simulink model "EST_Modified_Copy"  (R2023a)
settings: Solver=FixedStepAuto  StartTime=0.0  StopTime=stopt  FixedStep=deltat  MaxStep=0.05  RelTol=1e-3
InitFcn:
  | clear all;
  | close all;
  | clc;
  | 
  | % add the data and script directories
  | addpath('data','scripts');
  | 
  | % load the constants (units)
  | constants;
  | 
  | % load the simulation parameters
  | preprocessing;
StopFcn:
  | postprocessing;
values from neighbouring files (symbols this model uses):
  aDemandTransport = 0.03    [preprocessing.m]
  aExtraction = 0.80    (= 0.8)    [preprocessing.m]
  aHeatCompressor = 0.07    [preprocessing.m]
  aHeatGenerator = 0.1    [preprocessing.m]
  aInjection = 0.15    [preprocessing.m]
  aSupplyTransport = 0.03    [preprocessing.m]
  bHeatExchanger = 0.001    [preprocessing.m]
  bStorage = 0.000/unit("s")    [preprocessing.m]
  EStorageInitial = 0.000*unit("kWh")    [preprocessing.m]
  EStorageMax = (25/3)*unit("kWh")    [preprocessing.m]
  EStorageMin = 0.000*unit("kWh")    [preprocessing.m]
  HeatExchangerInitial = 0    [preprocessing.m]
settings Model: Creator=joche  LastModifiedBy=20221247
settings DataIOCC: SaveFormat=Array  SaveOutput=off  ReturnWorkspaceOutputs=off
settings OptimizationCC: ReuseModelBlockBuffer=off
settings ModelReferenceCC: EnableRefExpFcnMdlSchedulingChecks=on

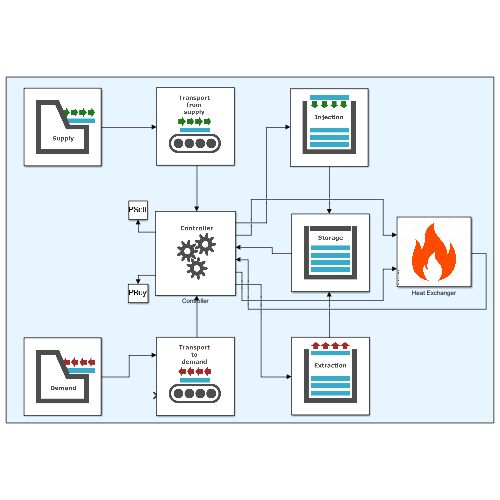
[thumbnail: Simulink's stored preview of the top-level diagram]
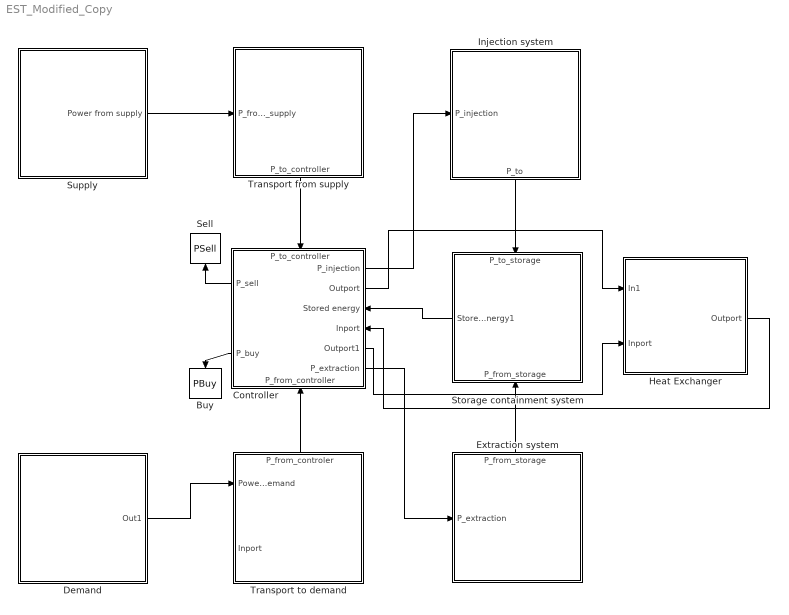
== system EST_Modified_Copy ==
  Buy : ToWorkspace  VariableName=PBuy  SampleTime=-1
  Controller : Subsystem
      settings: PortSchema="{\"entries\":[{\"content\":{\"sides\":[{\"content\":{\"connectorIds\":[\"Out5\",\"Out6\"]},\"type\":\"ConnectorPlacement.EquallySpacedRectSide\",\"uuid\":\"4daf33ce-c96a-4783-b5c4-228eed953e01\"},{\"content\":{\"connectorIds\":[\"Out1\",\"Out2\",\"In3\",\"In4\",\"Out3\",\"Out4\"],\"side\":\"RIGHT\"},\"type\":\"ConnectorPlacement.EquallySpacedRectSide\",\"uuid\":\"e9942e50-8467-4af8-b79b-80636cbc76e5\"},{\"content\":{\"connectorIds\":[\"In1\"],\"side\":\"TOP\"},\"type\":\"ConnectorPlacement.EquallySpacedRectSide\",\"uuid\":\"f315e931-d69b-4751-b712-f89c6c81baeb\"},{\"content\":{\"connectorIds\":[\"In2\"],\"side\":\"BOTTOM\"},\"type\":\"ConnectorPlacement.EquallySpacedRectSide\",\"uuid\":\"44715ee6-5cd5-4669-bcb9-5ed7c869bdb3\"}]},\"type\":\"ConnectorPlacement.EquallySpacedConnector\",\"uuid\":\"fff48899-944b-4064-b7d7-ecc12144fb48\"}],\"packageUris\":[\"http://schema.mathworks.com/mf0/Connector/R2020b\"],\"version\":\"1.0\"}"
      mask Display: image('$imagefile'); % Use "Edit Image" on toolstrip to change.
  Demand : Subsystem
      mask Display: image('$imagefile'); % Use "Edit Image" on toolstrip to change.
  Extraction system : Subsystem
      settings: PortSchema="{\"entries\":[{\"content\":{\"sides\":[{\"content\":{},\"type\":\"ConnectorPlacement.EquallySpacedRectSide\",\"uuid\":\"05c5933d-55fc-4e06-853f-fc26d42905f9\"},{\"content\":{\"connectorIds\":[\"In1\"],\"side\":\"RIGHT\"},\"type\":\"ConnectorPlacement.EquallySpacedRectSide\",\"uuid\":\"327426c5-31d5-498b-a2bd-83e49353408c\"},{\"content\":{\"side\":\"TOP\"},\"type\":\"ConnectorPlacement.EquallySpacedRectSide\",\"uuid\":\"55306cf3-a3de-4385-a5ae-b8600ecdd5a2\"},{\"content\":{\"connectorIds\":[\"Out1\"],\"side\":\"BOTTOM\"},\"type\":\"ConnectorPlacement.EquallySpacedRectSide\",\"uuid\":\"08fcc9c3-40d3-4ac6-b914-dfeef6039ffb\"}]},\"type\":\"ConnectorPlacement.EquallySpacedConnector\",\"uuid\":\"cb35d5ba-e8c6-462c-b7b2-fe8356d4b0a1\"}],\"packageUris\":[\"http://schema.mathworks.com/mf0/Connector/R2020b\"],\"version\":\"1.0\"}"
      mask Display: image('$imagefile'); % Use "Edit Image" on toolstrip to change.
  Heat Exchanger : Subsystem
      mask Display: image('Heat Exchanger Icon.jpg'); % Use "Edit Image" on toolstrip to change.
  Injection system : Subsystem
      settings: PortSchema="{\"entries\":[{\"content\":{\"sides\":[{\"content\":{},\"type\":\"ConnectorPlacement.EquallySpacedRectSide\",\"uuid\":\"05c5933d-55fc-4e06-853f-fc26d42905f9\"},{\"content\":{\"connectorIds\":[\"In1\"],\"side\":\"RIGHT\"},\"type\":\"ConnectorPlacement.EquallySpacedRectSide\",\"uuid\":\"327426c5-31d5-498b-a2bd-83e49353408c\"},{\"content\":{\"connectorIds\":[\"Out1\"],\"side\":\"TOP\"},\"type\":\"ConnectorPlacement.EquallySpacedRectSide\",\"uuid\":\"55306cf3-a3de-4385-a5ae-b8600ecdd5a2\"},{\"content\":{\"side\":\"BOTTOM\"},\"type\":\"ConnectorPlacement.EquallySpacedRectSide\",\"uuid\":\"08fcc9c3-40d3-4ac6-b914-dfeef6039ffb\"}]},\"type\":\"ConnectorPlacement.EquallySpacedConnector\",\"uuid\":\"cb35d5ba-e8c6-462c-b7b2-fe8356d4b0a1\"}],\"packageUris\":[\"http://schema.mathworks.com/mf0/Connector/R2020b\"],\"version\":\"1.0\"}"
      mask Display: image('$imagefile'); % Use "Edit Image" on toolstrip to change.
  Sell : ToWorkspace  VariableName=PSell  SampleTime=-1
  Storage containment system : Subsystem
      settings: PortSchema="{\"entries\":[{\"content\":{\"sides\":[{\"content\":{\"connectorIds\":[\"Out1\"]},\"type\":\"ConnectorPlacement.EquallySpacedRectSide\",\"uuid\":\"0ba48424-33b9-4934-970f-64fe5d8b070e\"},{\"content\":{\"connectorIds\":[],\"side\":\"RIGHT\"},\"type\":\"ConnectorPlacement.EquallySpacedRectSide\",\"uuid\":\"9cde340f-8f39-4499-9a12-5e1623737660\"},{\"content\":{\"connectorIds\":[\"In1\"],\"side\":\"TOP\"},\"type\":\"ConnectorPlacement.EquallySpacedRectSide\",\"uuid\":\"2af8db04-7fd0-4902-8637-8dc00edb4598\"},{\"content\":{\"connectorIds\":[\"In2\"],\"side\":\"BOTTOM\"},\"type\":\"ConnectorPlacement.EquallySpacedRectSide\",\"uuid\":\"e21ea806-d777-41a3-a53f-556fae66854b\"}]},\"type\":\"ConnectorPlacement.EquallySpacedConnector\",\"uuid\":\"4e2ddb36-4db3-4ab4-858b-ebb8ccefeb1f\"}],\"packageUris\":[\"http://schema.mathworks.com/mf0/Connector/R2020b\"],\"version\":\"1.0\"}"
      mask Display: image('$imagefile'); % Use "Edit Image" on toolstrip to change.
  Supply : Subsystem
      mask Display: image('$imagefile'); % Use "Edit Image" on toolstrip to change.
  Transport from supply : Subsystem
      settings: PortSchema="{\"entries\":[{\"content\":{\"sides\":[{\"content\":{\"connectorIds\":[\"In1\"]},\"type\":\"ConnectorPlacement.EquallySpacedRectSide\",\"uuid\":\"31329006-3d36-4d93-9c44-7503a515d397\"},{\"content\":{\"connectorIds\":[],\"side\":\"RIGHT\"},\"type\":\"ConnectorPlacement.EquallySpacedRectSide\",\"uuid\":\"aba139c7-f9b6-4881-a56b-a4cbbedacd88\"},{\"content\":{\"connectorIds\":[],\"side\":\"TOP\"},\"type\":\"ConnectorPlacement.EquallySpacedRectSide\",\"uuid\":\"e683eb73-7a35-4160-9c39-da83856a6278\"},{\"content\":{\"connectorIds\":[\"Out1\"],\"side\":\"BOTTOM\"},\"type\":\"ConnectorPlacement.EquallySpacedRectSide\",\"uuid\":\"1170dd18-447c-437f-9043-6812c2877331\"}]},\"type\":\"ConnectorPlacement.EquallySpacedConnector\",\"uuid\":\"804af608-1d70-444f-af69-e05f19bf98f3\"}],\"packageUris\":[\"http://schema.mathworks.com/mf0/Connector/R2020b\"],\"version\":\"1.0\"}"
      mask Display: image('$imagefile'); % Use "Edit Image" on toolstrip to change.
  Transport to demand : Subsystem
      settings: PortSchema="{\"entries\":[{\"content\":{\"sides\":[{\"content\":{\"connectorIds\":[\"In1\",\"In2\"]},\"type\":\"ConnectorPlacement.EquallySpacedRectSide\",\"uuid\":\"31329006-3d36-4d93-9c44-7503a515d397\"},{\"content\":{\"side\":\"RIGHT\"},\"type\":\"ConnectorPlacement.EquallySpacedRectSide\",\"uuid\":\"aba139c7-f9b6-4881-a56b-a4cbbedacd88\"},{\"content\":{\"connectorIds\":[\"Out1\"],\"side\":\"TOP\"},\"type\":\"ConnectorPlacement.EquallySpacedRectSide\",\"uuid\":\"e683eb73-7a35-4160-9c39-da83856a6278\"},{\"content\":{\"side\":\"BOTTOM\"},\"type\":\"ConnectorPlacement.EquallySpacedRectSide\",\"uuid\":\"c378138f-7233-4483-870c-40a69b3495ee\"}]},\"type\":\"ConnectorPlacement.EquallySpacedConnector\",\"uuid\":\"804af608-1d70-444f-af69-e05f19bf98f3\"}],\"packageUris\":[\"http://schema.mathworks.com/mf0/Connector/R2020b\"],\"version\":\"1.0\"}"
      mask Display: image('$imagefile'); % Use "Edit Image" on toolstrip to change.
  wires:
  Supply/1(Power from supply) -> Transport from supply/1(P_from_supply)
  Transport from supply/1(P_to_controller) -> Controller/1(P_to_controller)
  Transport to demand/1(P_from_controler) -> Controller/2(P_from_controller)
  Demand/1(Out1) -> Transport to demand/1(Power to demand)
  Controller/5(P_sell) -> Sell/1
  Controller/4(P_extraction) -> Extraction system/1(P_extraction)
  Injection system/1(P_to) -> Storage containment system/1(P_to_storage)
  Extraction system/1(P_from_storage) -> Storage containment system/2(P_from_storage)
  Storage containment system/1(Stored energy1) -> Controller/3(Stored energy)
  Controller/1(P_injection) -> Injection system/1(P_injection)
  Controller/6(P_buy) -> Buy/1
  Controller/2(Outport) -> Heat Exchanger/1(In1)
  Controller/3(Outport1) -> Heat Exchanger/2(Inport)
  Heat Exchanger/1(Outport) -> Controller/4(Inport)

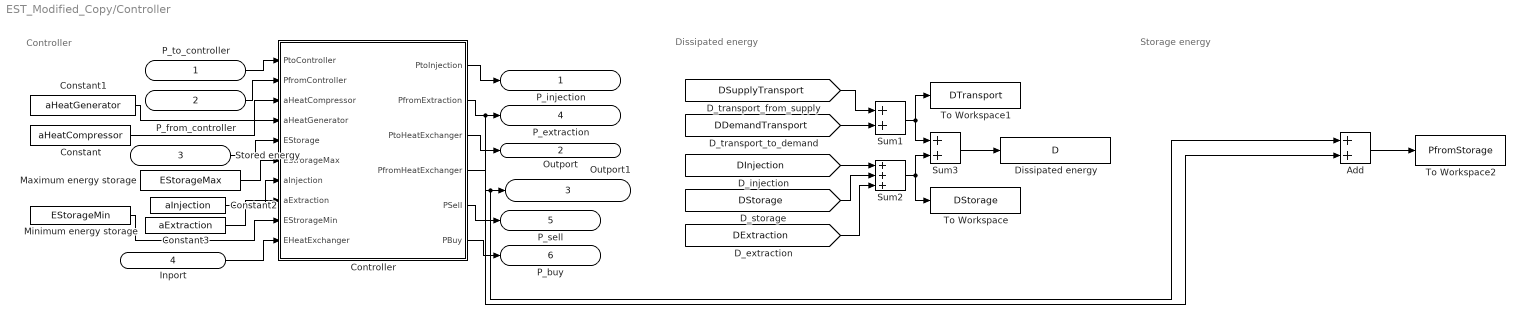
== system EST_Modified_Copy/Controller ==
  note: Dissipated energy
  note: Controller
  note: Storage energy
  P_to_controller : Inport
  P_from_controller : Inport  Port=2
  Stored energy : Inport  Port=3
  Inport : Inport  Port=4
  Add : Sum
  Constant : Constant  Value=aHeatCompressor
  Constant1 : Constant  Value=aHeatGenerator
  Constant2 : Constant  Value=aInjection
  Constant3 : Constant  Value=aExtraction
  Controller : MATLAB Function  TreatAsAtomicUnit=on
  Dissipated energy : ToWorkspace  VariableName=D  SampleTime=-1
  Maximum energy storage : Constant  Value=EStorageMax
  Minimum energy storage : Constant  Value=EStorageMin
  Sum1 : Sum
  Sum2 : Sum  Inputs=+++
  Sum3 : Sum
  To Workspace : ToWorkspace  VariableName=DStorage  SampleTime=-1
  To Workspace1 : ToWorkspace  VariableName=DTransport  SampleTime=-1
  To Workspace2 : ToWorkspace  VariableName=PfromStorage  SaveFormat=Timeseries  SampleTime=-1
  P_injection : Outport
  Outport : Outport  Port=2
  Outport1 : Outport  Port=3
  P_extraction : Outport  Port=4
  P_sell : Outport  Port=5
  P_buy : Outport  Port=6
  wires:
  P_from_controller/1 -> Controller/2(PfromController)
  Controller/5(PSell) -> P_sell/1
  Controller/6(PBuy) -> P_buy/1
  Minimum energy storage/1 -> Controller/9(EStrorageMin)
  Maximum energy storage/1 -> Controller/6(EStrorageMax)
  P_to_controller/1 -> Controller/1(PtoController)
  Controller/1(PtoInjection) -> P_injection/1
  Stored energy/1 -> Controller/5(EStorage)
  [DDemandTransport] -> Sum1/2
  [DSupplyTransport] -> Sum1/1
  [DInjection] -> Sum2/1
  [DStorage] -> Sum2/2
  [DExtraction] -> Sum2/3
  Sum2/1 -> To Workspace/1, Sum3/2
  Sum1/1 -> To Workspace1/1, Sum3/1
  Sum3/1 -> Dissipated energy/1
  Controller/3(PtoHeatExchanger) -> Outport/1
  Constant/1 -> Controller/3(aHeatCompressor)
  Constant2/1 -> Controller/7(aInjection)
  Constant3/1 -> Controller/8(aExtraction)
  Inport/1 -> Controller/10(EHeatExchanger)
  Controller/4(PfromHeatExchanger) -> Add/1, Outport1/1
  Controller/2(PfromExtraction) -> Add/2, P_extraction/1
  Add/1 -> To Workspace2/1
  Constant1/1 -> Controller/4(aHeatGenerator)

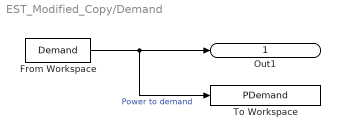
== system EST_Modified_Copy/Demand ==
  From Workspace : FromWorkspace  VariableName=Demand  Interpolate=off  OutputAfterFinalValue=Setting to zero
  To Workspace : ToWorkspace  VariableName=PDemand  SampleTime=-1
  Out1 : Outport
  wires:
  From Workspace/1 -> To Workspace/1, Out1/1  "Power to demand"

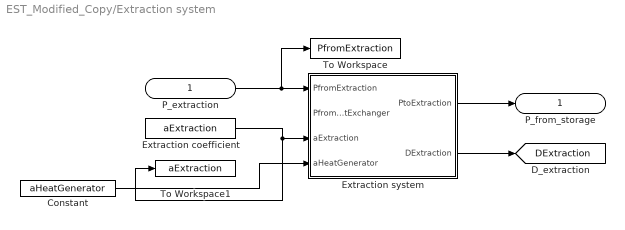
== system EST_Modified_Copy/Extraction system ==
  P_extraction : Inport
  Constant : Constant  Value=aHeatGenerator
  Extraction coefficient : Constant  Value=aExtraction
  Extraction system : MATLAB Function  TreatAsAtomicUnit=on
  To Workspace : ToWorkspace  VariableName=PfromExtraction  SampleTime=-1
  To Workspace1 : ToWorkspace  VariableName=aExtraction  SaveFormat=Timeseries  SampleTime=-1
  P_from_storage : Outport
  tag scope: DExtraction=global
  wires:
  P_extraction/1 -> Extraction system/1(PfromExtraction), To Workspace/1
  Extraction system/1(PtoExtraction) -> P_from_storage/1
  Extraction coefficient/1 -> To Workspace1/1, Extraction system/3(aExtraction)
  Extraction system/2(DExtraction) -> [DExtraction]
  Constant/1 -> Extraction system/4(aHeatGenerator)

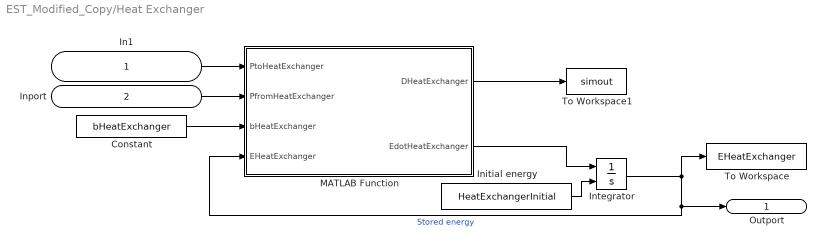
== system EST_Modified_Copy/Heat Exchanger ==
  In1 : Inport
  Inport : Inport  Port=2
  Constant : Constant  Value=bHeatExchanger
  Initial energy : Constant  Value=HeatExchangerInitial
  Integrator : Integrator  InitialConditionSource=external  LimitOutput=on  UpperSaturationLimit=EStorageMax  LowerSaturationLimit=EStorageMin
  MATLAB Function : MATLAB Function  TreatAsAtomicUnit=on
  To Workspace : ToWorkspace  VariableName=EHeatExchanger  SampleTime=-1
  To Workspace1 : ToWorkspace  VariableName=simout  SaveFormat=Timeseries  SampleTime=-1
  Outport : Outport
  wires:
  In1/1 -> MATLAB Function/1(PtoHeatExchanger)
  MATLAB Function/1(DHeatExchanger) -> To Workspace1/1
  Constant/1 -> MATLAB Function/3(bHeatExchanger)
  Integrator/1 -> Outport/1, MATLAB Function/4(EHeatExchanger), To Workspace/1  "Stored energy"
  Initial energy/1 -> Integrator/2
  MATLAB Function/2(EdotHeatExchanger) -> Integrator/1
  Inport/1 -> MATLAB Function/2(PfromHeatExchanger)

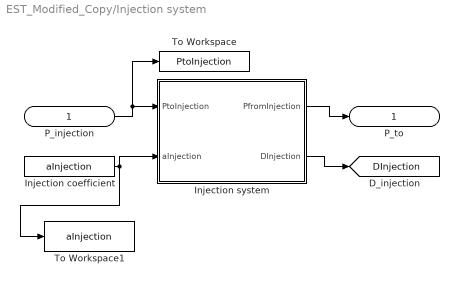
== system EST_Modified_Copy/Injection system ==
  P_injection : Inport
  Injection coefficient : Constant  Value=aInjection
  Injection system : MATLAB Function  TreatAsAtomicUnit=on
  To Workspace : ToWorkspace  VariableName=PtoInjection  SampleTime=-1
  To Workspace1 : ToWorkspace  VariableName=aInjection  SaveFormat=Timeseries  SampleTime=-1
  P_to : Outport
  tag scope: DInjection=global
  wires:
  P_injection/1 -> To Workspace/1, Injection system/1(PtoInjection)
  Injection system/1(PfromInjection) -> P_to/1
  Injection coefficient/1 -> To Workspace1/1, Injection system/2(aInjection)
  Injection system/2(DInjection) -> [DInjection]

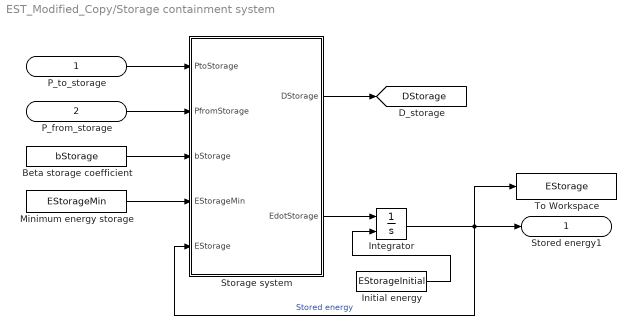
== system EST_Modified_Copy/Storage containment system ==
  P_to_storage : Inport
  P_from_storage : Inport  Port=2
  Beta storage coefficient : Constant  Value=bStorage
  Initial energy : Constant  Value=EStorageInitial
  Integrator : Integrator  InitialConditionSource=external  LimitOutput=on  UpperSaturationLimit=EStorageMax  LowerSaturationLimit=EStorageMin
  Minimum energy storage : Constant  Value=EStorageMin
  Storage system : MATLAB Function  TreatAsAtomicUnit=on
  To Workspace : ToWorkspace  VariableName=EStorage  SampleTime=-1
  Stored energy1 : Outport
  tag scope: DStorage=global
  wires:
  P_from_storage/1 -> Storage system/2(PfromStorage)
  P_to_storage/1 -> Storage system/1(PtoStorage)
  Initial energy/1 -> Integrator/2
  Integrator/1 -> To Workspace/1, Storage system/5(EStorage), Stored energy1/1  "Stored energy"
  Storage system/1(DStorage) -> [DStorage]
  Beta storage coefficient/1 -> Storage system/3(bStorage)
  Storage system/2(EdotStorage) -> Integrator/1
  Minimum energy storage/1 -> Storage system/4(EStorageMin)

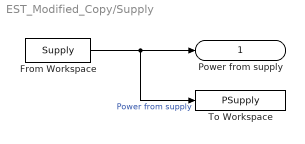
== system EST_Modified_Copy/Supply ==
  From Workspace : FromWorkspace  VariableName=Supply  Interpolate=off  OutputAfterFinalValue=Setting to zero
  To Workspace : ToWorkspace  VariableName=PSupply  SampleTime=-1
  Power from supply : Outport
  wires:
  From Workspace/1 -> To Workspace/1, Power from supply/1  "Power from supply"

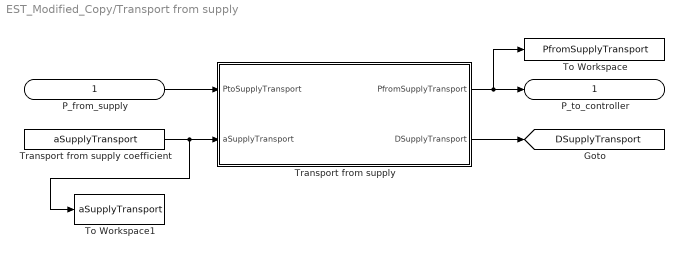
== system EST_Modified_Copy/Transport from supply ==
  P_from_supply : Inport
  To Workspace : ToWorkspace  VariableName=PfromSupplyTransport  SampleTime=-1
  To Workspace1 : ToWorkspace  VariableName=aSupplyTransport  SaveFormat=Timeseries  SampleTime=-1
  Transport from supply : MATLAB Function  TreatAsAtomicUnit=on
  Transport from supply coefficient : Constant  Value=aSupplyTransport
  P_to_controller : Outport
  tag scope: DSupplyTransport=global
  wires:
  Transport from supply coefficient/1 -> To Workspace1/1, Transport from supply/2(aSupplyTransport)
  P_from_supply/1 -> Transport from supply/1(PtoSupplyTransport)
  Transport from supply/1(PfromSupplyTransport) -> To Workspace/1, P_to_controller/1
  Transport from supply/2(DSupplyTransport) -> [DSupplyTransport]

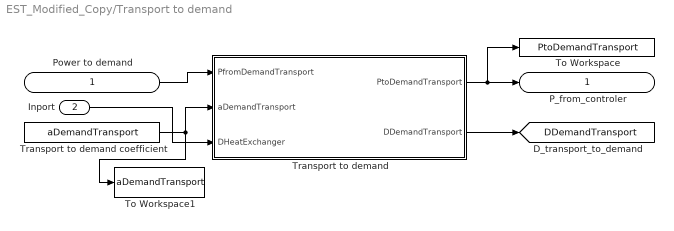
== system EST_Modified_Copy/Transport to demand ==
  Power to demand : Inport
  Inport : Inport  Port=2
  To Workspace : ToWorkspace  VariableName=PtoDemandTransport  SampleTime=-1
  To Workspace1 : ToWorkspace  VariableName=aDemandTransport  SaveFormat=Timeseries  SampleTime=-1
  Transport to demand : MATLAB Function  TreatAsAtomicUnit=on
  Transport to demand coefficient : Constant  Value=aDemandTransport
  P_from_controler : Outport
  tag scope: DDemandTransport=global
  wires:
  Transport to demand coefficient/1 -> To Workspace1/1, Transport to demand/2(aDemandTransport)
  Power to demand/1 -> Transport to demand/1(PfromDemandTransport)
  Transport to demand/1(PtoDemandTransport) -> To Workspace/1, P_from_controler/1
  Transport to demand/2(DDemandTransport) -> [DDemandTransport]
  Inport/1 -> Transport to demand/3(DHeatExchanger)

== matlab function EST_Modified_Copy/Heat Exchanger/MATLAB Function ==
  data: PtoHeatExchanger input; PfromHeatExchanger input; DHeatExchanger output; bHeatExchanger input; EdotHeatExchanger output; EHeatExchanger input
function [DHeatExchanger, EdotHeatExchanger] = HeatExchanger(PtoHeatExchanger, PfromHeatExchanger, bHeatExchanger, EHeatExchanger)
DHeatExchanger = bHeatExchanger * EHeatExchanger;
EdotHeatExchanger = PtoHeatExchanger - PfromHeatExchanger - DHeatExchanger;

== matlab function EST_Modified_Copy/Transport to demand/Transport to demand ==
  data: PfromDemandTransport input; PtoDemandTransport output; aDemandTransport input; DDemandTransport output; DHeatExchanger input
% function [PtoDemandTransport, DDemandTransport] = demandTransport(PfromDemandTransport, aDemandTransport)
%     DDemandTransport = 1 / (1 - aDemandTransport) * PfromDemandTransport;   % modified line
% 
%     %calculating losses in inverter
%     PtoDemandTransportAfterInverter = PfromDemandTransport * (1 - aDemandTransport);
% 
%     %Losses in wire (this calculation is dynamic) (P^2/V^2 * R)
%     R = 0.0000000168 * (DemandWireLength/0.0000125633);
%     WireLoss = ((PtoDemandTransportAfterInverter^2 / 230^2) *  R);
% 
%     %Add to the output values
%     DDemandTransport = WireLoss;
%     PtoDemandTransport = PfromDemandTransport + DDemandTransport;

function [PtoDemandTransport, DDemandTransport] = demandTransport(PfromDemandTransport, aDemandTransport, DHeatExchanger)

    %aSupplyTransport the Dissipation caused by the inverter
    DemandWireLength = 15;

    %calculating losses in inverter
    PtoDemandTransportAfterInverter = PfromDemandTransport * (1 - aDemandTransport);

    %Losses in wire (this calculation is dynamic) (P^2/V^2 * R)
    R = 0.0000000168 * (DemandWireLength/0.0000125633);
    WireLoss = ((PtoDemandTransportAfterInverter^2 / 230^2) *  R);

    %Add to the output values
    DDemandTransport = WireLoss;
    PtoDemandTransport = PfromDemandTransport + DDemandTransport + DHeatExchanger;

== matlab function EST_Modified_Copy/Injection system/Injection system ==
  data: PtoInjection input; PfromInjection output; aInjection input; DInjection output
function [PfromInjection, DInjection] = injection(PtoInjection, aInjection)
    % Perhaps function[PtoHeatExchanger] = injection(aHeatCompressor)

    DInjection = aInjection * PtoInjection;
    PfromInjection = PtoInjection - DInjection; % Power from injector is supplied as the difference between Power generated and the efficiency of the compressor.

    % PtoHeatExchanger = aHeatCompressor * PtoInjection;  % Power that is transferred as heat to the heat exchanger.

== matlab function EST_Modified_Copy/Transport from supply/Transport from supply ==
  data: PtoSupplyTransport input; PfromSupplyTransport output; aSupplyTransport input; DSupplyTransport output
% function [PfromSupplyTransport, DSupplyTransport] = supplyTransport(PtoSupplyTransport, aSupplyTransport)
%     DSupplyTransport = aSupplyTransport * PtoSupplyTransport;
%     PfromSupplyTransport = PtoSupplyTransport - DSupplyTransport;

function [PfromSupplyTransport, DSupplyTransport] = supplyTransport(PtoSupplyTransport, aSupplyTransport)

%This should be moved to the Preproccsing matlab script
SupplyWireLength = 20;


%aSupplyTransport the Dissipation caused by the inverter

%calculating losses in inverter
PtoSupplyTransportAfterInverter = PtoSupplyTransport * (1 - aSupplyTransport);

%Losses in wire (this calculation is dynamic) (P^2/V^2 * R)
R = 0.0000000168 * (SupplyWireLength/0.0000125633);
WireLoss = ((PtoSupplyTransportAfterInverter^2 / 230^2) *  R);

%Add to the output values
DSupplyTransport = WireLoss;
PfromSupplyTransport = PtoSupplyTransportAfterInverter - DSupplyTransport; 

%  if(WireLoss ~= 0)
%  disp(WireLoss * 100 / PtoSupplyTransport)
%  disp(DSupplyTransport)
%  PfromSupplyTransport
%  end


%   DSupplyTransport = PtoSupplyTransport * aSupplyTransport;
%   PfromSupplyTransport = PtoSupplyTransport - DSupplyTransport;

== matlab function EST_Modified_Copy/Controller/Controller ==
  data: PtoInjection output; PfromExtraction output; PtoHeatExchanger output; PfromHeatExchanger output; PSell output; PBuy output; PtoController input; PfromController input; aHeatCompressor input; aHeatGenerator input; EStorage input; EStrorageMax input; aInjection input; aExtraction input; EStrorageMin input; EHeatExchanger input
function [PtoInjection, PfromExtraction, PtoHeatExchanger, PfromHeatExchanger, PSell, PBuy] = controller(PtoController, PfromController, aHeatCompressor, aHeatGenerator, EStorage, EStrorageMax, aInjection, aExtraction, EStrorageMin, EHeatExchanger)
% Perhaps function[... PtoHeatExchanger, PfromHeatExchanger] =
% controller(aHeatGenerator, aHeatCompressor);

    %% Power surplus or deficit

    deltaP = PtoController - PfromController;

    PtoHeatExchanger = 0;
    PfromHeatExchanger = 0;

    % Power surplus
    if deltaP >= 0

        %% Storage injection

        % Storage system is not full
        if EStorage < EStrorageMax 

            PtoInjection = deltaP * (1 - aInjection);
            PtoHeatExchanger = deltaP * aHeatCompressor;

        % Storage system is full
        else
            PtoInjection = 0;
            PtoHeatExchanger = 0;
        end

        %% Storage extraction

        PfromExtraction = 0;

        %% Load-balancing
        PSell   = deltaP - PtoInjection - PtoHeatExchanger;
        PBuy    = 0;

    % Power deficit
    else

        %% Storage injection

        PtoInjection = 0;

        %% Storage extraction

        % Storage system is not empty
        if EStorage > EStrorageMin

            PfromExtraction = -deltaP * (aExtraction);

                if EHeatExchanger > 0
                    PfromHeatExchanger = (-deltaP - PfromExtraction) * aHeatGenerator;

                else
                    PfromHeatExchanger = 0;
                end


        % Storage system is empty
        else
            PfromExtraction = 0;
            PfromHeatExchanger = 0;
        end

        %% Load-balancing

        PSell = 0;
        PBuy  = -deltaP - PfromExtraction - PfromHeatExchanger;
    end

== matlab function EST_Modified_Copy/Extraction system/Extraction system ==
  data: PfromExtraction input; PfromHeatExchanger input; PtoExtraction output; aExtraction input; DExtraction output; aHeatGenerator input
function [PtoExtraction, DExtraction] = extraction(PfromExtraction, PfromHeatExchanger, aExtraction, aHeatGenerator)
% Perhaps function [] = extraction(PfromHeatExchanger, aHeatGenerator)

    DExtraction = 1 / (aExtraction) * PfromExtraction;  % modified line
    DHeatExchanger = PfromHeatExchanger * aHeatGenerator;
    PtoExtraction = DExtraction + DHeatExchanger;  % modified line

== matlab function EST_Modified_Copy/Storage containment system/Storage system ==
  data: DStorage output; EdotStorage output; PtoStorage input; PfromStorage input; bStorage input; EStorageMin input; EStorage input
function [DStorage, EdotStorage]= Storage(PtoStorage, PfromStorage, bStorage, EStorageMin, EStorage)
    DStorage = bStorage * (EStorage-EStorageMin);
    EdotStorage = PtoStorage - PfromStorage - DStorage;
